simulink model "addr"  (Simulink 7.8)
settings: Solver=FixedStepDiscrete  StartTime=0.0  StopTime=10.0  RelTol=1e-3
libraries: rappid_ec_lib x13, simulink x6, rappid_lib x1
settings Model: Creator=Embed_Sys_course  LastModifiedBy=Embed_Sys_course
settings DataIOCC: ExternalInput=off  InitialState=off  SaveOutput=off  SignalLogging=off  SaveTime=off
settings OptimizationCC: InlineParams=on  OptimizeModelRefInitCode=on  LifeSpan=1
settings DebuggingCC: InheritedTsInSrcMsg=none  SingleTaskRateTransMsg=error  UnderSpecifiedDataTypeMsg=error  UnnecessaryDatatypeConvMsg=warning  UnconnectedInputMsg=error  UnconnectedOutputMsg=error  UnconnectedLineMsg=error  UnknownTsInhSupMsg=error
settings HardwareCC: ProdLargestAtomicInteger=Long  ProdLargestAtomicFloat=Double  ProdIntDivRoundTo=Zero  ProdEndianess=BigEndian  ProdHWDeviceType=Motorola PowerPC
settings RTWCC: SystemTargetFile=rappid.tlc  MakeCommand=rappid_make_rtw  TemplateMakefile=rappid_default_tmf  PostCodeGenCommand=rappid_analyzegencode(buildInfo)  Description=RAppID Toolbox MPC5554 Code Generation Target (rappid)  ProcessScript=rappid_make_rtw_hook
settings CodeAppCC: IgnoreCustomStorageClasses=off
settings STFCustomTargetCC: ModelReferenceCompliant=off  GeneratePreprocessorConditionals=Use local settings  CombineOutputUpdateFcns=on  ERTCustomFileBanners=on  SupportContinuousTime=off  SupportNonInlinedSFcns=off  SystemTargetFile=rappid.tlc
settings ERTTargetCC: MultiwordLength=2048  ModelReferenceCompliant=off  ParMdlRefBuildCompliant=off  CompOptLevelCompliant=off  ConcurrentExecutionCompliant=off  ERTFirstTimeCompliant=off  ModelStepFunctionPrototypeControlCompliant=off  CPPClassGenCompliant=off  InlinedParameterPlacement=NonHierarchical  ERTCustomFileTemplate=example_file_process.tlc  ConvertIfToSwitch=off  SuppressUnreachableDefaultCases=off

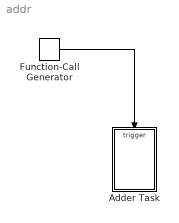
== system addr ==
  Adder Task : Subsystem
  Function-Call Generator : simulink/Ports & Subsystems/Function-Call Generator  sample_time=0.1  numberOfIterations=1
  wires:
  Function-Call Generator/1 -> Adder Task/Trigger

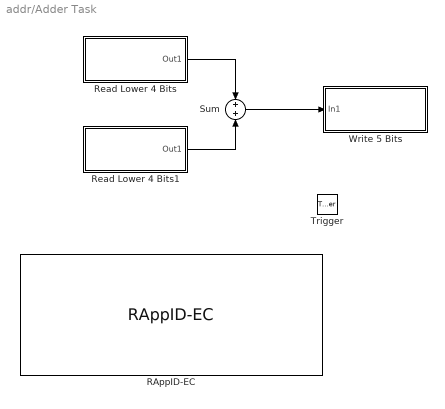
== system addr/Adder Task ==
  Trigger : TriggerPort  TriggerType=function-call  PortDimensions=1
  RAppID-EC : rappid_lib/RAppID Initialization Blocks/RAppID-EC  Tag=RAppID  Priority=0  rtos=simpletarget  targetmcu=IntRAM  clockfrequency=128  basetaskpriority=20  systemcounter=0  systimer_isrpriority=1  systimer_period=0  isrstacksize=50  interruptdispatcher=None  stored_mdl_name=addr
  Read Lower 4 Bits : Subsystem
  Read Lower 4 Bits1 : Subsystem
  Sum : Sum
  Write 5 Bits : Subsystem
  wires:
  Sum/1 -> Write 5 Bits/1(In1)
  Read Lower 4 Bits1/1(Out1) -> Sum/2
  Read Lower 4 Bits/1(Out1) -> Sum/1

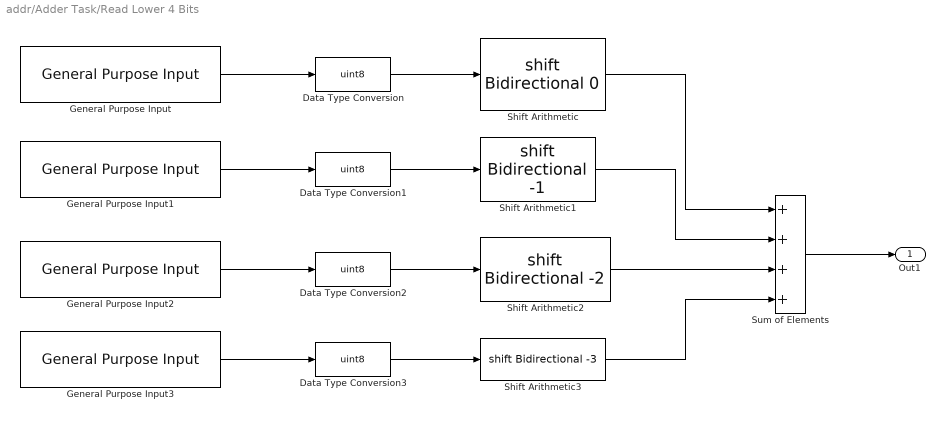
== system addr/Adder Task/Read Lower 4 Bits ==
  Data Type Conversion{,1..3} (4 alike) : DataTypeConversion  OutDataTypeStr=uint8
  General Purpose Input : rappid_ec_lib/Peripheral Driver Blocks/GPIO Blocks/General Purpose Input  gpoi_inputs="93:   Primary Function \"DSPI SCKA\""  pinNum=93
  General Purpose Input1 : rappid_ec_lib/Peripheral Driver Blocks/GPIO Blocks/General Purpose Input  gpoi_inputs="94:   Primary Function \"DSPI SINA\""  pinNum=94
  General Purpose Input2 : rappid_ec_lib/Peripheral Driver Blocks/GPIO Blocks/General Purpose Input  gpoi_inputs="95:   Primary Function \"DSPI SOUTA\""  pinNum=95
  General Purpose Input3 : rappid_ec_lib/Peripheral Driver Blocks/GPIO Blocks/General Purpose Input  gpoi_inputs="96:   Primary Function \"DSPI PCSA0\""  pinNum=96
  Shift Arithmetic : ArithShift
  Shift Arithmetic1 : ArithShift  BitShiftNumber=-1
  Shift Arithmetic2 : ArithShift  BitShiftNumber=-2
  Shift Arithmetic3 : ArithShift  BitShiftNumber=-3
  Sum of Elements : Sum  Inputs=++++  AccumDataTypeStr=uint8
  Out1 : Outport
  wires:
  Sum of Elements/1 -> Out1/1
  Data Type Conversion/1 -> Shift Arithmetic/1
  Data Type Conversion1/1 -> Shift Arithmetic1/1
  Data Type Conversion2/1 -> Shift Arithmetic2/1
  Data Type Conversion3/1 -> Shift Arithmetic3/1
  Shift Arithmetic/1 -> Sum of Elements/1
  Shift Arithmetic1/1 -> Sum of Elements/2
  Shift Arithmetic2/1 -> Sum of Elements/3
  Shift Arithmetic3/1 -> Sum of Elements/4
  General Purpose Input/1 -> Data Type Conversion/1
  General Purpose Input1/1 -> Data Type Conversion1/1
  General Purpose Input2/1 -> Data Type Conversion2/1
  General Purpose Input3/1 -> Data Type Conversion3/1

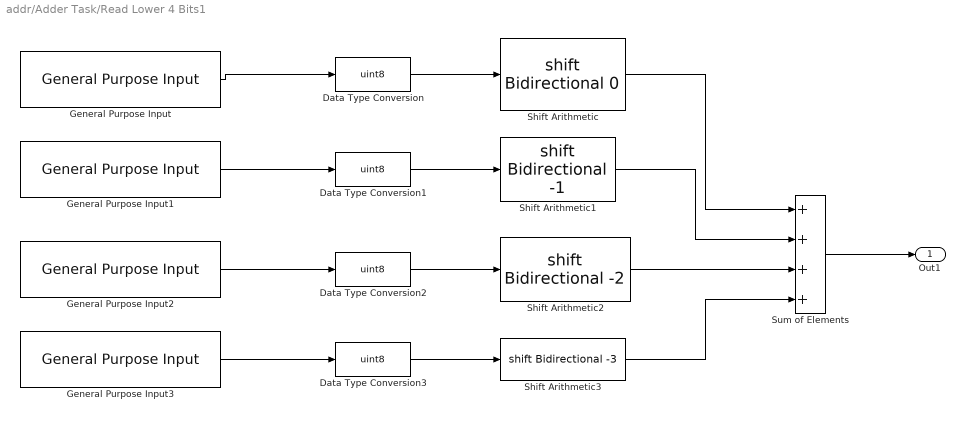
== system addr/Adder Task/Read Lower 4 Bits1 ==
  Data Type Conversion{,1..3} (4 alike) : DataTypeConversion  OutDataTypeStr=uint8
  General Purpose Input : rappid_ec_lib/Peripheral Driver Blocks/GPIO Blocks/General Purpose Input  gpoi_inputs="97:   Primary Function \"DSPI PCSA1\""  pinNum=97
  General Purpose Input1 : rappid_ec_lib/Peripheral Driver Blocks/GPIO Blocks/General Purpose Input  gpoi_inputs="98:   Primary Function \"DSPI PCSA2\""  pinNum=98
  General Purpose Input2 : rappid_ec_lib/Peripheral Driver Blocks/GPIO Blocks/General Purpose Input  gpoi_inputs="99:   Primary Function \"DSPI PCSA3\""  pinNum=99
  General Purpose Input3 : rappid_ec_lib/Peripheral Driver Blocks/GPIO Blocks/General Purpose Input  gpoi_inputs="100:   Primary Function \"DSPI PCSA4\""  pinNum=100
  Shift Arithmetic : ArithShift
  Shift Arithmetic1 : ArithShift  BitShiftNumber=-1
  Shift Arithmetic2 : ArithShift  BitShiftNumber=-2
  Shift Arithmetic3 : ArithShift  BitShiftNumber=-3
  Sum of Elements : Sum  Inputs=++++  AccumDataTypeStr=uint8
  Out1 : Outport
  wires:
  Sum of Elements/1 -> Out1/1
  Data Type Conversion/1 -> Shift Arithmetic/1
  Data Type Conversion1/1 -> Shift Arithmetic1/1
  Data Type Conversion2/1 -> Shift Arithmetic2/1
  Data Type Conversion3/1 -> Shift Arithmetic3/1
  Shift Arithmetic/1 -> Sum of Elements/1
  Shift Arithmetic1/1 -> Sum of Elements/2
  Shift Arithmetic2/1 -> Sum of Elements/3
  Shift Arithmetic3/1 -> Sum of Elements/4
  General Purpose Input/1 -> Data Type Conversion/1
  General Purpose Input1/1 -> Data Type Conversion1/1
  General Purpose Input2/1 -> Data Type Conversion2/1
  General Purpose Input3/1 -> Data Type Conversion3/1

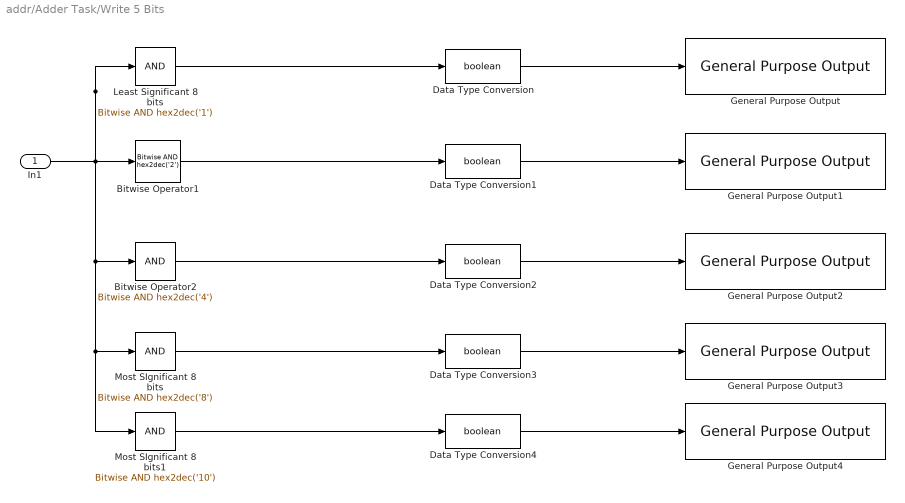
== system addr/Adder Task/Write 5 Bits ==
  In1 : Inport  OutDataTypeStr=uint8
  Bitwise Operator1 : simulink/Logic and Bit Operations/Bitwise Operator  logicop=AND  UseBitMask=on  BitMask=hex2dec('2')  BitMaskRealWorld=Stored Integer
  Bitwise Operator2 : simulink/Logic and Bit Operations/Bitwise Operator  logicop=AND  UseBitMask=on  BitMask=hex2dec('4')  BitMaskRealWorld=Stored Integer
  Data Type Conversion{,1..4} (5 alike) : DataTypeConversion  OutDataTypeStr=boolean  LockScale=on
  General Purpose Output : rappid_ec_lib/Peripheral Driver Blocks/GPIO Blocks/General Purpose Output  gpoi_outputs="101:   Primary Function \"DSPI PCSA5\""  pinNum=101
  General Purpose Output1 : rappid_ec_lib/Peripheral Driver Blocks/GPIO Blocks/General Purpose Output  gpoi_outputs="102:   Primary Function \"DSPI SCKB\""  pinNum=102
  General Purpose Output2 : rappid_ec_lib/Peripheral Driver Blocks/GPIO Blocks/General Purpose Output  gpoi_outputs="103:   Primary Function \"DSPI SINB\""  pinNum=103
  General Purpose Output3 : rappid_ec_lib/Peripheral Driver Blocks/GPIO Blocks/General Purpose Output  gpoi_outputs="104:   Primary Function \"DSPI SOUTB\""  pinNum=104
  General Purpose Output4 : rappid_ec_lib/Peripheral Driver Blocks/GPIO Blocks/General Purpose Output  gpoi_outputs="105:   Primary Function \"DSPI PCSB0\""  pinNum=105
  Least Significant 8 bits : simulink/Logic and Bit Operations/Bitwise Operator  logicop=AND  UseBitMask=on  BitMask=hex2dec('1')  BitMaskRealWorld=Stored Integer
  Most SIgnificant 8 bits : simulink/Logic and Bit Operations/Bitwise Operator  logicop=AND  UseBitMask=on  BitMask=hex2dec('8')  BitMaskRealWorld=Stored Integer
  Most SIgnificant 8 bits1 : simulink/Logic and Bit Operations/Bitwise Operator  logicop=AND  UseBitMask=on  BitMask=hex2dec('10')  BitMaskRealWorld=Stored Integer
  wires:
  In1/1 -> Least Significant 8 bits/1, Bitwise Operator1/1, Bitwise Operator2/1, Most SIgnificant 8 bits/1, Most SIgnificant 8 bits1/1
  Most SIgnificant 8 bits1/1 -> Data Type Conversion4/1
  Most SIgnificant 8 bits/1 -> Data Type Conversion3/1
  Bitwise Operator2/1 -> Data Type Conversion2/1
  Bitwise Operator1/1 -> Data Type Conversion1/1
  Least Significant 8 bits/1 -> Data Type Conversion/1
  Data Type Conversion/1 -> General Purpose Output/1
  Data Type Conversion1/1 -> General Purpose Output1/1
  Data Type Conversion2/1 -> General Purpose Output2/1
  Data Type Conversion3/1 -> General Purpose Output3/1
  Data Type Conversion4/1 -> General Purpose Output4/1
